simulink library "compelx_real_2c4t_lib"  (Simulink 8.7)
settings: Solver=ode45  StartTime=0.0  StopTime=10.0  RelTol=1e-3
undefined symbols (not defined in the file): AdvDSPBChannelOutDisplay, CFR_LINEUP_param, dpoly, dspba_ChannelInVis, dspba_ChannelOutVis, dspba_internal_get_channel_ports, dspba_internal_get_demux_ports, evalAionMaskParam, latency, primtype, value
libraries: DSPBAPrim x17, Pipereg_lib x2, DSPBABase x1
settings Model: Creator=bigcat  LastModifiedBy=5g

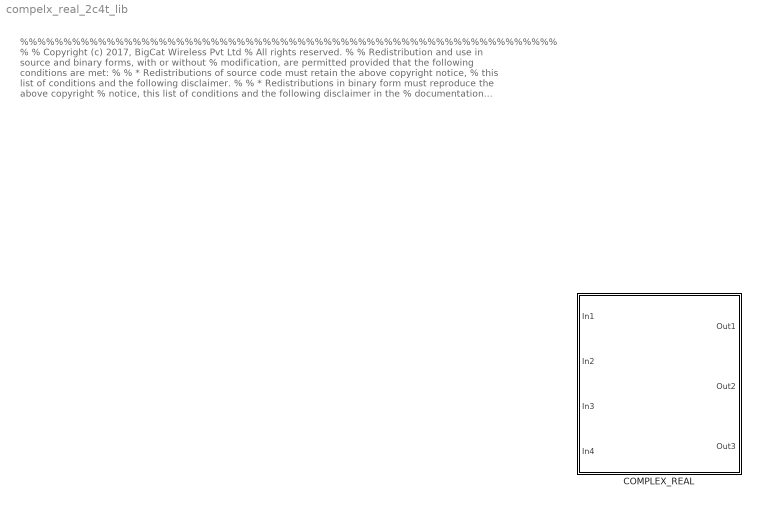
== system compelx_real_2c4t_lib ==
  note: %%%%%%%%%%%%%%%%%%%%%%%%%%%%%%%%%%%%%%%%%%%%%%%%%%%%%%%%%%%%%%
      |  %
      |  % Copyright (c) 2017, BigCat Wireless Pvt Ltd
      |  % All rights reserved.
      |  %
      |  % Redistribution and use in source and binary forms, with or without
      |  % modification, are permitted provided that the following conditions are met:
      |  %
      |  %     * Redistributions of source code must retain the above copyright notice,
      |  %       this list of conditions and the following disclaimer.
      |  %
      |  %     * Redistributions in binary form must reproduce the above copyright
      |  %       notice, this list of conditions and the following disclaimer in the
      |  %       documentation and/or other materials provided with the distribution.
      |  %
      |  %     * Neither the name of the copyright holder nor the names of its contributors
      |  %       may be used to endorse or promote products derived from this software
      |  %       without specific prior written permission.
      |  %
      |  %
      |  %
      |  % THIS SOFTWARE IS PROVIDED BY THE COPYRIGHT HOLDERS AND CONTRIBUTORS "AS IS"
      |  % AND ANY EXPRESS OR IMPLIED WARRANTIES, INCLUDING, BUT NOT LIMITED TO, THE
      |  % IMPLIED WARRANTIES OF MERCHANTABILITY AND FITNESS FOR A PARTICULAR PURPOSE ARE
      |  % DISCLAIMED. IN NO EVENT SHALL THE COPYRIGHT HOLDER OR CONTRIBUTORS BE LIABLE
      |  % FOR ANY DIRECT, INDIRECT, INCIDENTAL, SPECIAL, EXEMPLARY, OR CONSEQUENTIAL
      |  % DAMAGES (INCLUDING, BUT NOT LIMITED TO, PROCUREMENT OF SUBSTITUTE GOODS OR
      |  % SERVICES; LOSS OF USE, DATA, OR PROFITS; OR BUSINESS INTERRUPTION) HOWEVER
      |  % CAUSED AND ON ANY THEORY OF LIABILITY, WHETHER IN CONTRACT, STRICT LIABILITY,
      |  % OR TORT (INCLUDING NEGLIGENCE OR OTHERWISE) ARISING IN ANY WAY OUT OF THE USE
      |  % OF THIS SOFTWARE, EVEN IF ADVISED OF THE POSSIBILITY OF SUCH DAMAGE.
      |  %
      |   %%%%%%%%%%%%%%%%%%%%%%%%%%%%%%%%%%%%%%%%%%%%%%%%%%%%%%%%%%%%%
  COMPLEX_REAL : Subsystem  mask{Latency=20, ClockMargin=CFR_LINEUP_param.ClockMargin_DUC, Pipeline_stages=2}
      mask Display:
      | disp('COMPLEX_REAL');
      | port_label('input',3,'v');
      | port_label('input',4,'c');
      | port_label('input',1,'d0');
      | port_label('input',2,'d0');
      | port_label('output',2,'q_v');
      | port_label('output',3,'q_c');
      | port_label('output',1,'q');

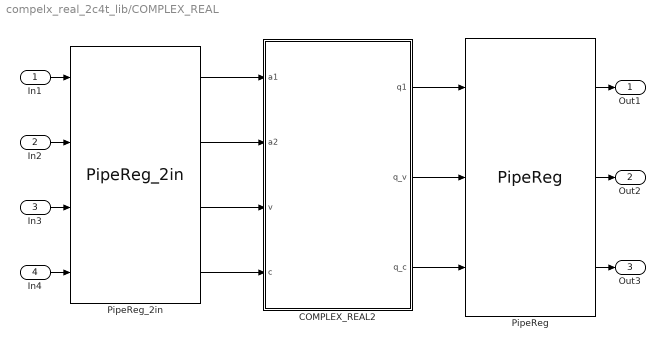
== system compelx_real_2c4t_lib/COMPLEX_REAL ==
  In1 : Inport
  In2 : Inport  Port=2
  In3 : Inport  Port=3
  In4 : Inport  Port=4
  COMPLEX_REAL2 : Subsystem
  PipeReg : Pipereg_lib/PipeReg  NPipe=Pipeline_stages  Clock_Margin=ClockMargin
  PipeReg_2in : Pipereg_lib/PipeReg_2in  NPipe=Pipeline_stages  Clock_Margin=ClockMargin
  Out1 : Outport
  Out2 : Outport  Port=2
  Out3 : Outport  Port=3
  wires:
  PipeReg/1 -> Out1/1
  PipeReg/3 -> Out3/1
  COMPLEX_REAL2/1(q1) -> PipeReg/1
  PipeReg_2in/1 -> COMPLEX_REAL2/1(a1)
  PipeReg_2in/2 -> COMPLEX_REAL2/2(a2)
  PipeReg/2 -> Out2/1
  In3/1 -> PipeReg_2in/3
  COMPLEX_REAL2/3(q_c) -> PipeReg/3
  COMPLEX_REAL2/2(q_v) -> PipeReg/2
  In2/1 -> PipeReg_2in/2
  PipeReg_2in/3 -> COMPLEX_REAL2/3(v)
  In4/1 -> PipeReg_2in/4
  PipeReg_2in/4 -> COMPLEX_REAL2/4(c)
  In1/1 -> PipeReg_2in/1

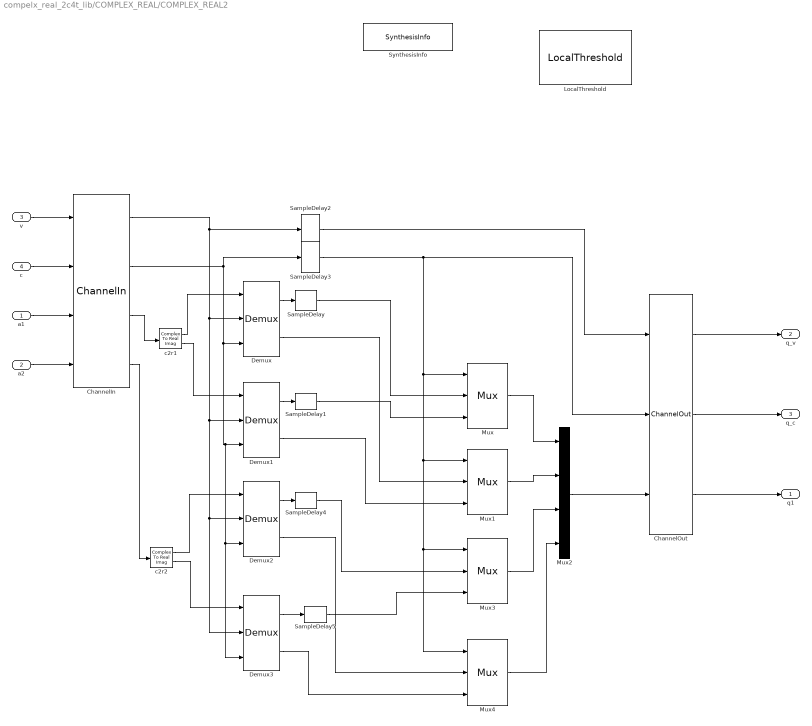
== system compelx_real_2c4t_lib/COMPLEX_REAL/COMPLEX_REAL2 ==
  a1 : Inport
  a2 : Inport  Port=2
  v : Inport  Port=3
  c : Inport  Port=4
  ChannelIn : DSPBAPrim/ChannelIn  primtype=channelin  nInputs=dspba_internal_get_channel_ports(gcb)  nOutputs=dspba_internal_get_channel_ports(gcb)  omode=Inherit via internal rule  otype=sfix(16)  scale=2^-15  rndmethod=Unbiased  factor=1  satmethod=Symmetric  shift_vec=[0 1 2 -1]  value=2  inPortNames=['v'; 'c'; '0'; '1'; '2'; '3'; '4'; '5'; '6'; '7'; '8'; '9'; 'A'; 'B'; 'D'; 'E'; 'F'; 'G'; 'H'; 'I'; 'J'; 'K'; 'L'; 'M'; 'N'; 'O'; 'P'; 'Q'; 'R'; 'S'; 'T'; 'U'; 'W'; 'X'; 'Y'; 'Z']  outPortNames=['v'; 'c'; '0'; '1'; '2'; '3'; '4'; '5'; '6'; '7'; '8'; '9'; 'A'; 'B'; 'D'; 'E'; 'F'; 'G'; 'H'; 'I'; 'J'; 'K'; 'L'; 'M'; 'N'; 'O'; 'P'; 'Q'; 'R'; 'S'; 'T'; 'U'; 'W'; 'X'; 'Y'; 'Z']  dspbaimage=dspba_prim.jpg  text=fprintf('In');  style=Optimised  dataSignals=2  foldingEnabled=off  channels=1  sampleRate=200  packetBeginPresent=off  packetBeginEnabled=off  visibilities=dspba_ChannelInVis(gcb)  latencyCorrection=0  version=20141013
  ChannelOut : DSPBAPrim/ChannelOut  primtype=channelout  nInputs=dspba_internal_get_channel_ports(gcb)  nOutputs=dspba_internal_get_channel_ports(gcb)  omode=Inherit via internal rule  otype=sfix(16)  scale=2^-15  rndmethod=Unbiased  factor=1  satmethod=Symmetric  shift_vec=[0 1 2 -1]  value=1  inPortNames=['v'; 'c'; '0'; '1'; '2'; '3'; '4'; '5'; '6'; '7'; '8'; '9'; 'A'; 'B'; 'D'; 'E'; 'F'; 'G'; 'H'; 'I'; 'J'; 'K'; 'L'; 'M'; 'N'; 'O'; 'P'; 'Q'; 'R'; 'S'; 'T'; 'U'; 'W'; 'X'; 'Y'; 'Z']  outPortNames=['v'; 'c'; '0'; '1'; '2'; '3'; '4'; '5'; '6'; '7'; '8'; '9'; 'A'; 'B'; 'D'; 'E'; 'F'; 'G'; 'H'; 'I'; 'J'; 'K'; 'L'; 'M'; 'N'; 'O'; 'P'; 'Q'; 'R'; 'S'; 'T'; 'U'; 'W'; 'X'; 'Y'; 'Z']  dspbaimage=dspba_prim.jpg  text=fprintf('Out%s', AdvDSPBChannelOutDisplay(latency));  style=Optimised  dataSignals=1  foldingEnabled=off  channels=1  sampleRate=200  packetBeginPresent=off  packetBeginEnabled=off  visibilities=dspba_ChannelOutVis(gcb)  latency=21  latencyCorrection=0  version=20141013
  Demux{,1..3} (4 alike) : DSPBAPrim/Demux  primtype=demux  nInputs=3  nOutputs=dspba_internal_get_demux_ports(gcb)  omode=Inherit via internal rule  otype=sfix(16)  scale=2^-15  rndmethod=Unbiased  factor=1  satmethod=Symmetric  shift_vec=[0 1]  value=2  inPortNames=['q'; 'v'; 'c']  outPortNames=['c0'; 'c1']  dspbaimage=dspba_prim.jpg  text=fprintf('demux');  style=Optimised  visibilities=1536  version=20100120
  LocalThreshold : DSPBABase/LocalThreshold  margin=ClockMargin  delayRegOrRAMThresholdBits=10000  MediumDualMemThresholdBits=10000  LargeDualMemThresholdBits=-1  hardMultiplierThresholdLuts=-1  version=0
  Mux{,1,3..4} (4 alike) : DSPBAPrim/Mux  primtype=mux  nInputs=evalAionMaskParam(gcb,'value',1)+1  nOutputs=1  omode=Inherit via internal rule  otype=sfix(16)  scale=2^-15  rndmethod=Unbiased  factor=1  satmethod=Symmetric  shift_vec=[0 1 2 -1]  value=2  inPortNames=['s '; 'd0'; 'd1'; 'd2'; 'd3'; 'd4'; 'd5'; 'd6'; 'd7'; 'd8'; 'd9';]  outPortNames=[' ']  dspbaimage=dspba_prim.jpg  text=fprintf('%s', primtype);  style=Optimised  visibilities=1032  version=20131025
  Mux2 : Mux
  SampleDelay{,1..5} (6 alike) : DSPBAPrim/SampleDelay  primtype=sampdelay  nInputs=1  nOutputs=1  omode=Inherit via internal rule  otype=sfix(16)  scale=2^-15  rndmethod=Unbiased  factor=1  satmethod=Symmetric  shift_vec=[0 1 2 -1]  value=1  inPortNames=[' '; ' ';]  outPortNames=[' ']  dspbaimage=dspba_prim.jpg  text=dpoly(1, eye(1,value+1), 'z')  style=Optimised  visibilities=8 + 1024 + 2^17 + 2^18  flexible=off  slackgroup=0  augmented=0  version=20090407  advOptions=[]
  SynthesisInfo : DSPBAPrim/SynthesisInfo  primtype=synthinfo  nInputs=0  nOutputs=0  omode=Inherit via internal rule  otype=sfix(16)  scale=2^-15  rndmethod=Truncate  factor=1  satmethod=Symmetric  shift_vec=[0 1 2 -1]  value=99  inPortNames=[' '; ' ';]  outPortNames=[' ']  dspbaimage=dspba_prim_ctrl.jpg  text=fprintf('Style=%s', style);  style=Scheduled  visibilities=2^15+2^17+2^18+2^19  constraintInUse=on  constraintRelation=>  constraintLimit=Latency  bitAccurate=off  version=20090407
  c2r1 : ComplexToRealImag
  c2r2 : ComplexToRealImag
  q1 : Outport
  q_v : Outport  Port=2
  q_c : Outport  Port=3
  wires:
  Mux4/1 -> Mux2/4
  Mux3/1 -> Mux2/3
  Demux3/2 -> Mux4/3
  Demux2/2 -> Mux4/2
  SampleDelay5/1 -> Mux3/3
  Demux3/1 -> SampleDelay5/1
  SampleDelay4/1 -> Mux3/2
  Demux2/1 -> SampleDelay4/1
  c2r2/2 -> Demux3/1
  c2r2/1 -> Demux2/1
  ChannelIn/4 -> c2r2/1
  a2/1 -> ChannelIn/4
  Mux1/1 -> Mux2/2
  Mux/1 -> Mux2/1
  SampleDelay3/1 -> ChannelOut/2, Mux1/1, Mux4/1, Mux3/1, Mux/1
  SampleDelay2/1 -> ChannelOut/1
  Mux2/1 -> ChannelOut/3
  Demux1/2 -> Mux1/3
  Demux/2 -> Mux1/2
  SampleDelay1/1 -> Mux/3
  SampleDelay/1 -> Mux/2
  Demux1/1 -> SampleDelay1/1
  Demux/1 -> SampleDelay/1
  ChannelIn/2 -> Demux1/3, Demux3/3, Demux2/3, Demux/3, SampleDelay3/1
  c2r1/2 -> Demux1/1
  c2r1/1 -> Demux/1
  ChannelIn/1 -> Demux1/2, Demux3/2, Demux2/2, Demux/2, SampleDelay2/1
  ChannelIn/3 -> c2r1/1
  c/1 -> ChannelIn/2
  ChannelOut/3 -> q1/1
  ChannelOut/2 -> q_c/1
  v/1 -> ChannelIn/1
  ChannelOut/1 -> q_v/1
  a1/1 -> ChannelIn/3
